simulink model "TesteSimulVR"  (R2017a)
settings: Solver=VariableStepAuto  StartTime=0.0  StopTime=50  RelTol=1e-3
values from neighbouring files (symbols this model uses):
  IN = h(:,1)    [ImportData.m]
  OUT = h(:,2)    [ImportData.m]
libraries: vrlib x2, shared3dof x1, simulink x1
settings Model: Creator=Pichau  LastModifiedBy=Pichau

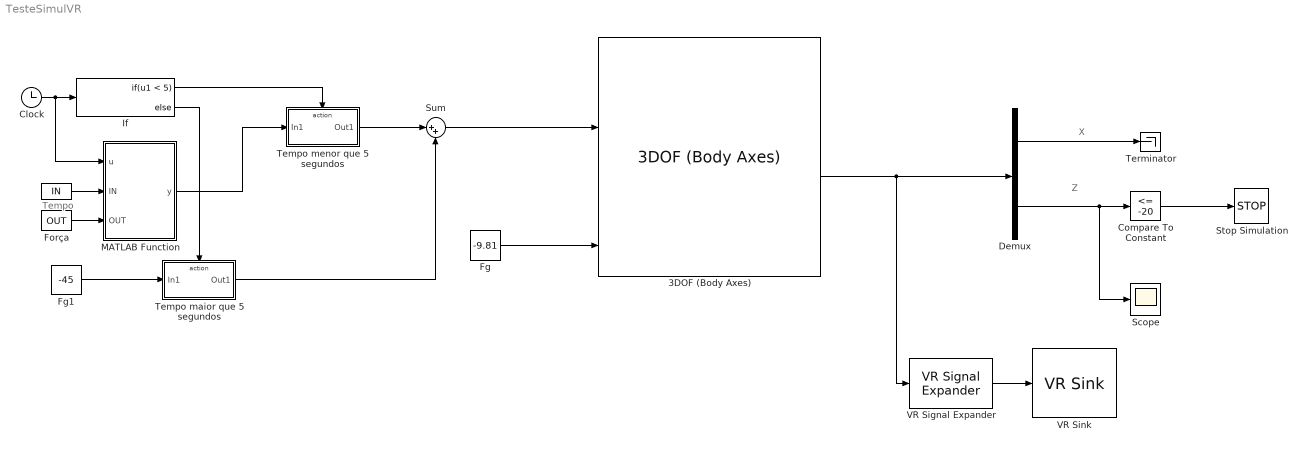
== system TesteSimulVR ==
  note: Tempo
  note: Z
  note: X
  " " : Constant  Value=IN
  3DOF (Body Axes) : shared3dof/3DOF (Body Axes)  units=Metric (MKS)  mtype=Fixed  v_ini=0  theta_ini=0  alpha_ini=0  q_ini=0  pos_ini=[0 0]  mass=1.0  mass_e=0.5  mass_f=3.0  Iyy=1.0  Iyy_e=0.5  Iyy_f=3.0  g_in=External  g=9.81  vre_flag=on  abi_flag=off
  Clock : Clock
  Compare To Constant : simulink/Logic and Bit Operations/Compare To Constant  relop=<=  const=-20  OutDataTypeStr=boolean
  Demux : Demux  Outputs=2
  Fg : Constant  Value=-9.81
  "Fg1 " : Constant  Value=-45
  Força : Constant  Value=OUT
  If : If  IfExpression=u1 < 5
  MATLAB Function : MATLAB Function  TreatAsAtomicUnit=on
  Scope : Scope
  Stop Simulation : Stop
  Sum : Sum  Inputs=|++
  Tempo maior que 5 segundos : Subsystem  TreatAsAtomicUnit=on
  Tempo menor que 5 segundos : Subsystem  TreatAsAtomicUnit=on
  Terminator : Terminator
  VR Signal Expander : vrlib/VR Signal Expander  outwidth=3  outidx=[1 2]
      settings: SourceProductName=Simulink 3D Animation  SourceProductBaseCode=VR
  VR Sink : vrlib/VR Sink  InstantiateOnLoad=on  SampleTime=0.02  ViewEnable=on  RemoteChange=off  RemoteView=off  FieldsWritten=Foguete.translation.3.1.1.double  WorldFileName=foguete.wrl  AutoView=off  VideoDimensions=[]  AllowVariableSize=off
      settings: SourceProductBaseCode=VR
  wires:
  Clock/1 -> MATLAB Function/1(u), If/1
  If/2 -> Tempo maior que 5 segundos/Action
  If/1 -> Tempo menor que 5 segundos/Action
  "Fg1 "/1 -> Tempo maior que 5 segundos/1(In1)
  Tempo menor que 5 segundos/1(Out1) -> Sum/1
  Tempo maior que 5 segundos/1(Out1) -> Sum/2
  Sum/1 -> 3DOF (Body Axes)/2
  Fg/1 -> 3DOF (Body Axes)/4
  3DOF (Body Axes)/4 -> VR Signal Expander/1, Demux/1
  Demux/1 -> Terminator/1
  Demux/2 -> Scope/1, Compare To Constant/1
  Compare To Constant/1 -> Stop Simulation/1
  MATLAB Function/1(y) -> Tempo menor que 5 segundos/1(In1)
  " "/1 -> MATLAB Function/2(IN)
  Força/1 -> MATLAB Function/3(OUT)
  VR Signal Expander/1 -> VR Sink/1

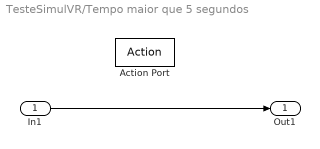
== system TesteSimulVR/Tempo maior que 5 segundos ==
  In1 : Inport
  Action Port : ActionPort  ActionType=else
  Out1 : Outport
  wires:
  In1/1 -> Out1/1

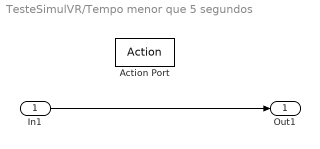
== system TesteSimulVR/Tempo menor que 5 segundos ==
  In1 : Inport
  Action Port : ActionPort  ActionType=then
  Out1 : Outport
  wires:
  In1/1 -> Out1/1

== matlab function TesteSimulVR/MATLAB Function ==
  data: u input; y output; IN input; OUT input
function y = fcn(u,IN,OUT)

y = interp1(IN,OUT,u);

end
